simulink model "vexarmcortex_BEST_IR_Sensor_Encoder"  (R2019a)
settings: Solver=FixedStepAuto  StartTime=0.0  StopTime=inf  RelTol=1e-3  EnableMultiTasking=on
libraries: vexarmcortexlib x4, simulink x1
settings Model: ExtModeTrigDuration=25  Creator=The MathWorks, Inc.  LastModifiedBy=josea
settings DataIOCC: ReturnWorkspaceOutputs=off
settings OptimizationCC: MaxStackSize=64
settings DebuggingCC: ParameterTunabilityLossMsg=error  ArithmeticOperatorsInVariantConditions=warning
settings HardwareCC: ProdBitPerPointer=32  ProdBitPerSizeT=32  ProdBitPerPtrDiffT=32  ProdLargestAtomicInteger=Long  ProdLargestAtomicFloat=Double  ProdWordSize=32  ProdHWDeviceType=ARM Compatible->ARM Cortex  UseEmbeddedCoderFeatures=off
settings SFSimCC: SimUseLocalCustomCode=off
settings RTWCC: SystemTargetFile=ert.tlc  HardwareBoard=ARM Cortex-based VEX Microcontroller  TLCOptions="-aInlineSetEventsForThisBaseRateFcn=TLC_FALSE -aSuppressMultiTaskScheduler=TLC_FALSE  -aRateBasedStepFcn=0"  TemplateMakefile=ert_default_tmf  RTWUseLocalCustomCode=off  Toolchain=GNU Tools for VEX ARM Cortex
settings CodeAppCC: ForceParamTrailComments=on  OperatorAnnotations=on  StateflowObjectComments=on  MATLABSourceComments=on
settings ERTTargetCC: ERTCustomFileBanners=off  SupportContinuousTime=on  SupportNonInlinedSFcns=on  RemoveResetFunc=off  ModelStepFunctionPrototypeControlCompliant=off

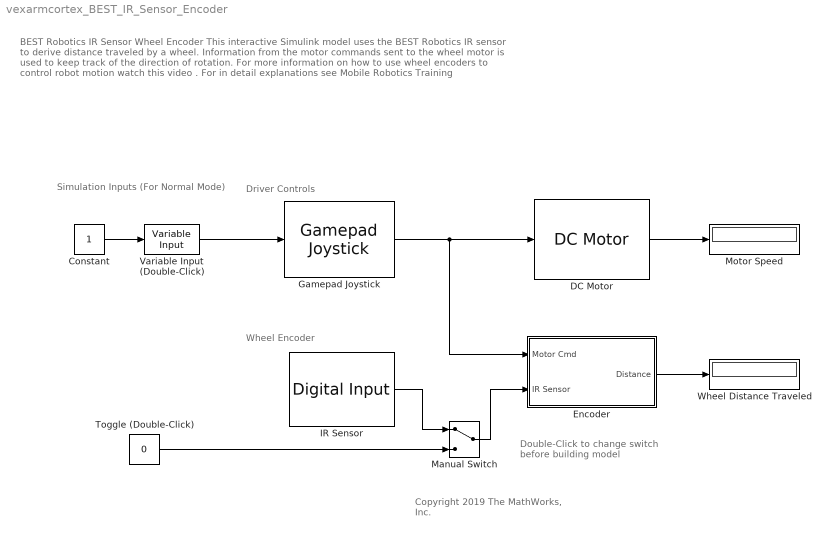
== system vexarmcortex_BEST_IR_Sensor_Encoder ==
  note: Double-Click to change switch
      | before building model
  note: Simulation Inputs
      | (For Normal Mode)
  note: Wheel Encoder
  note: Driver Controls
  note: BEST Robotics IR Sensor Wheel Encoder
      |
      | This interactive Simulink model uses the BEST Robotics IR sensor to derive distance traveled by a wheel.
      | Information from the motor commands sent to the wheel motor is used to keep track of the direction of rotation.
      | For more information on how to use wheel encoders to control robot motion watch this video .
      | For in detail explanations see Mobile Robotics Training
  note: Copyright 2019 The MathWorks, Inc.
  Constant : Constant
  DC Motor : vexarmcortexlib/Actuators/DC Motor  motor=1  scaleFactor=1/13.5  SimulationOut=on
      settings: SourceProductName=Simulink Coder Support Package for ARM Cortex-based VEX Microcontroller  SourceProductBaseCode=EC_VEX_MICRO
  Encoder : Subsystem
  Gamepad Joystick : vexarmcortexlib/Gamepad/Gamepad Joystick  joystick=1  chan=3  SimulationIn=on  SampleTime=0.02
      settings: SourceProductName=Simulink Coder Support Package for ARM Cortex-based VEX Microcontroller  SourceProductBaseCode=EC_VEX_MICRO
  IR Sensor : vexarmcortexlib/Sensors/Digital Input  inChan=3  SimulationIn=off  SampleTime=0.05
      settings: SourceProductName=Simulink Coder Support Package for ARM Cortex-based VEX Microcontroller  SourceProductBaseCode=EC_VEX_MICRO
  Manual Switch : ManualSwitch
  Motor Speed : Display
  Toggle (Double-Click) : Constant  Value=0
      settings: OpenFcn=|
      | if strcmp('0',get_param(gcb, 'Value'))                        set_param(gcb, 'Value', '1');
      | else
      |             set_param(gcb, 'Value', '0');
      | end
  Variable Input (Double-Click) : vexarmcortexlib/Utilities/Variable Input  low=-127  gain=0  high=127
      settings: SourceProductName=Simulink Coder Support Package for ARM Cortex-based VEX Microcontroller  SourceProductBaseCode=EC_VEX_MICRO
  Wheel Distance Traveled : Display
  wires:
  Encoder/1(Distance) -> Wheel Distance Traveled/1
  Gamepad Joystick/1 -> Encoder/1(Motor Cmd), DC Motor/1
  Variable Input (Double-Click)/1 -> Gamepad Joystick/1
  Constant/1 -> Variable Input (Double-Click)/1
  DC Motor/1 -> Motor Speed/1
  Toggle (Double-Click)/1 -> Manual Switch/2
  IR Sensor/1 -> Manual Switch/1
  Manual Switch/1 -> Encoder/2(IR Sensor)

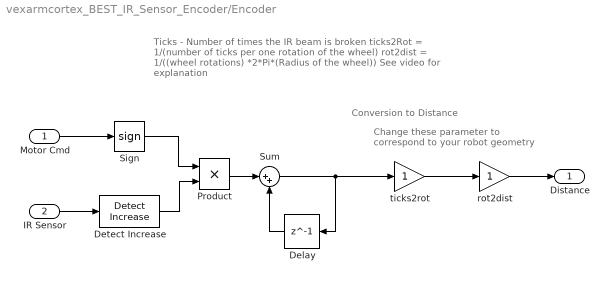
== system vexarmcortex_BEST_IR_Sensor_Encoder/Encoder ==
  note: Conversion to Distance
  note: Change these parameter to
      | correspond to your robot geometry
  note: Ticks - Number of times the IR beam is broken
      | ticks2Rot = 1/(number of ticks per one rotation of the wheel)
      | rot2dist = 1/((wheel rotations) *2*Pi*(Radius of the wheel))
      |
      | See video for explanation
  Motor Cmd : Inport
  IR Sensor : Inport  Port=2
  Delay : Delay  DelayLength=1
  Detect Increase : simulink/Logic and Bit Operations/Detect Increase  vinit=0.0  OutDataTypeStr=uint8
  Product : Product
  Sign : Signum
  Sum : Sum  Inputs=|++
  rot2dist : Gain
  ticks2rot : Gain
  Distance : Outport
  wires:
  IR Sensor/1 -> Detect Increase/1
  Sum/1 -> Delay/1, ticks2rot/1
  Delay/1 -> Sum/2
  Detect Increase/1 -> Product/2
  Product/1 -> Sum/1
  Motor Cmd/1 -> Sign/1
  Sign/1 -> Product/1
  ticks2rot/1 -> rot2dist/1
  rot2dist/1 -> Distance/1
